simulink model "pid_flc_steppermotor"  (R2014a)
settings: Solver=ode45  StartTime=0.0  StopTime=10  RelTol=1e-3
libraries: fuzblock x1
settings Model: Creator=KRISH  LastModifiedBy=krish
settings DebuggingCC: MaxConsecutiveZCsMsg=none  SolverPrmCheckMsg=none

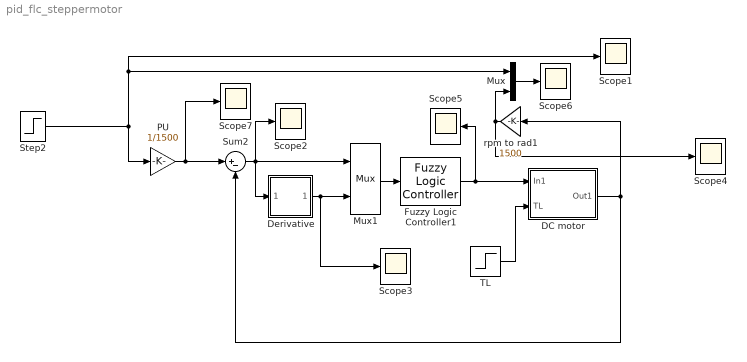
== system pid_flc_steppermotor ==
  DC motor : Subsystem  mask{Ra=0.05, La=0.1, J=0.1, D=10.91}
      mask prompts: Ra "Armature Resistance (Ra)"; La "Armature Inductance (La)"; J "Inertia (J)"; D "Damping (B)"
  Derivative : Subsystem
  Fuzzy Logic Controller1 : fuzblock/Fuzzy Logic  Controller  fis='flc_pid2.fis'
  Mux : Mux  Inputs=2
  Mux1 : Mux  Inputs=2
  PU : Gain  Gain=1/1500
  Scope{1..7} (7 alike) : Scope
      Scope1 settings: YMin=1377.5  YMax=1522.5
      Scope2 settings: YMin=0  YMax=1750
      Scope3 settings: YMin=-2e-08  YMax=1.5e-08  SaveName=ScopeData2
      Scope4 settings: YMin=80  YMax=112.5  SaveName=ScopeData3
      Scope5 settings: YMin=0.76  YMax=0.76  SaveName=ScopeData4
      Scope6 settings: YMin=0  YMax=1500  SaveName=ScopeData5
      Scope7 settings: YMin=0.918334  YMax=1.015  SaveName=ScopeData6
  Step2 : Step  Time=5  Before=800  After=1450  SampleTime=0.0001  VectorParams1D=off
  Sum2 : Sum  Inputs=|+-
  TL : Step  Time=7  Before=0.0001  After=0.002  SampleTime=0  VectorParams1D=off
  rpm to rad1 : Gain  Gain=1500
  wires:
  Sum2/1 -> Mux1/1, Derivative/1(in_1), Scope2/1
  DC motor/1(Out1) -> rpm to rad1/1, Sum2/2
  Fuzzy Logic Controller1/1 -> DC motor/1(In1), Scope5/1
  Mux1/1 -> Fuzzy Logic Controller1/1
  Derivative/1(out_1) -> Mux1/2, Scope3/1
  rpm to rad1/1 -> Scope4/1, Mux/2
  PU/1 -> Sum2/1, Scope7/1
  TL/1 -> DC motor/2(TL)
  Mux/1 -> Scope6/1
  Step2/1 -> PU/1, Scope1/1, Mux/1

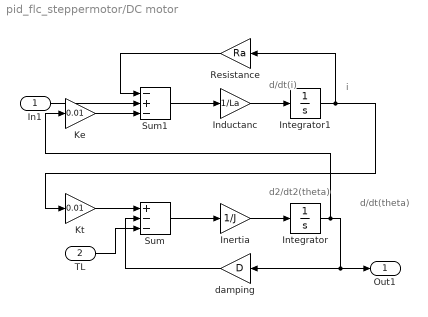
== system pid_flc_steppermotor/DC motor ==
  note: d/dt(i)
  note: i
  note: d/dt(theta)
  note: d2/dt2(theta)
  In1 : Inport
  TL : Inport  Port=2
  Inductanc : Gain  Gain=1/La  SaturateOnIntegerOverflow=on  OutDataTypeStr=Inherit: Same as input  ParamDataTypeStr=Inherit: Same as input
  Inertia : Gain  Gain=1/J  SaturateOnIntegerOverflow=on  OutDataTypeStr=Inherit: Same as input  ParamDataTypeStr=Inherit: Same as input
  Integrator : Integrator
  Integrator1 : Integrator
  Ke : Gain  Gain=0.01  SaturateOnIntegerOverflow=on  OutDataTypeStr=Inherit: Same as input  ParamDataTypeStr=Inherit: Same as input
  Kt : Gain  Gain=0.01  SaturateOnIntegerOverflow=on  OutDataTypeStr=Inherit: Same as input  ParamDataTypeStr=Inherit: Same as input
  Resistance : Gain  Gain=Ra  SaturateOnIntegerOverflow=on  OutDataTypeStr=Inherit: Same as input  ParamDataTypeStr=Inherit: Same as input
  Sum : Sum  Inputs=+--  SaturateOnIntegerOverflow=on  InputSameDT=on  OutDataTypeStr=Inherit: Same as first input
  Sum1 : Sum  Inputs=-+-  SaturateOnIntegerOverflow=on  InputSameDT=on  OutDataTypeStr=Inherit: Same as first input
  damping : Gain  Gain=D  SaturateOnIntegerOverflow=on  OutDataTypeStr=Inherit: Same as input  ParamDataTypeStr=Inherit: Same as input
  Out1 : Outport
  wires:
  Integrator1/1 -> Resistance/1, Kt/1
  Integrator/1 -> Ke/1, damping/1, Out1/1
  Ke/1 -> Sum1/3
  Resistance/1 -> Sum1/1
  Kt/1 -> Sum/1
  damping/1 -> Sum/2
  Sum1/1 -> Inductanc/1
  Sum/1 -> Inertia/1
  Inertia/1 -> Integrator/1
  Inductanc/1 -> Integrator1/1
  In1/1 -> Sum1/2
  TL/1 -> Sum/3

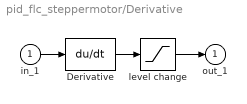
== system pid_flc_steppermotor/Derivative ==
  in_1 : Inport
  Derivative : Derivative
  level change : Saturate  UpperLimit=2  LowerLimit=-2
  out_1 : Outport
  wires:
  in_1/1 -> Derivative/1
  level change/1 -> out_1/1
  Derivative/1 -> level change/1
